simulink library "Counters_Lib"  (R2023a)
settings: Solver=ode45  StartTime=0.0  StopTime=10.0  RelTol=1e-3  EnableMultiTasking=on
libraries: simulink_extras x18, Miscellaneous x1
settings Model: Creator=Jozko Mrkvicka  LastModifiedBy=Jozko Mrkvicka
settings SolverCC: AlgebraicLoopSolver=TrustRegion
settings DataIOCC: LimitDataPoints=on  ReturnWorkspaceOutputs=off
settings OptimizationCC: LifeSpan=inf
settings DebuggingCC: UnconnectedInputMsg=warning  UnconnectedOutputMsg=warning  UnconnectedLineMsg=warning  AllowSymbolicDim=off  SFUnexpectedBacktrackingDiag=warning  SFNoUnconditionalDefaultTransitionDiag=warning  ArithmeticOperatorsInVariantConditions=warning
settings ModelReferenceCC: EnableRefExpFcnMdlSchedulingChecks=on
settings SFSimCC: SimUseLocalCustomCode=off  CustomCodeUndefinedFunction=UseInterfaceOnly
settings RTWCC: RTWUseLocalCustomCode=off
settings CodeAppCC: StateflowObjectComments=on
settings GRTTargetCC: TargetLangStandard=C89/C90 (ANSI)
settings ConfigComp: CovMetricSettings=dw  CovSaveCumulativeToWorkspaceVar=on  CovSaveSingleToWorkspaceVar=on  CovExternalEMLEnable=off

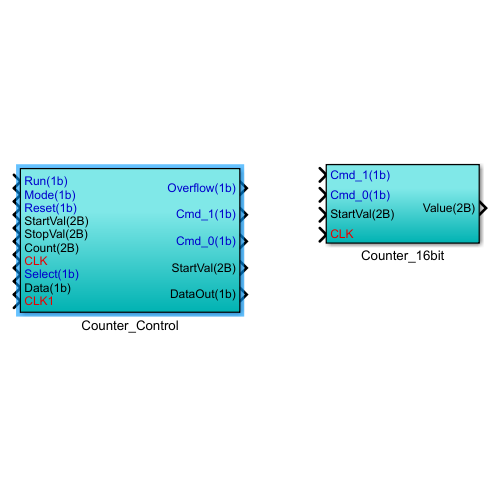
[thumbnail: Simulink's stored preview of the top-level diagram]
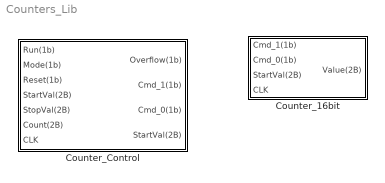
== system Counters_Lib ==
  Counter_16bit : Subsystem
  Counter_Control : Subsystem

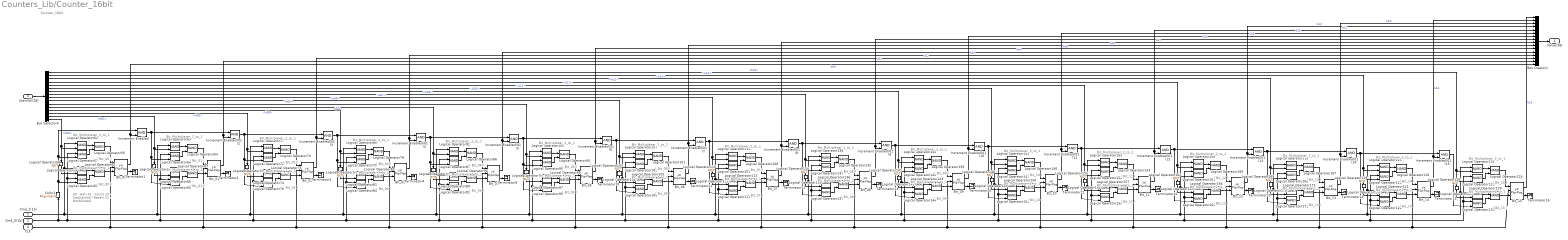
== system Counters_Lib/Counter_16bit ==
  note: Counter_16bit
  note: 00 - Halt
      | 01 - Count
      | 10 - SetStartVal (Reset)
      | 11 - NotAllowed
  note: ( Bit_00 )
  note: Bit_Multiplexer_2_to_1
  note: Bit_Multiplexer_2_to_1
  note: ( Bit_00 )
  note: ( Bit_01 )
  note: Bit_Multiplexer_2_to_1
  note: Bit_Multiplexer_2_to_1
  note: ( Bit_01 )
  note: ( Bit_02 )
  note: Bit_Multiplexer_2_to_1
  note: Bit_Multiplexer_2_to_1
  note: ( Bit_02 )
  note: ( Bit_03 )
  note: Bit_Multiplexer_2_to_1
  note: Bit_Multiplexer_2_to_1
  note: ( Bit_03 )
  note: ( Bit_04 )
  note: Bit_Multiplexer_2_to_1
  note: Bit_Multiplexer_2_to_1
  note: ( Bit_04 )
  note: ( Bit_05 )
  note: Bit_Multiplexer_2_to_1
  note: Bit_Multiplexer_2_to_1
  note: ( Bit_05 )
  note: ( Bit_06 )
  note: Bit_Multiplexer_2_to_1
  note: Bit_Multiplexer_2_to_1
  note: ( Bit_06 )
  note: ( Bit_07 )
  note: Bit_Multiplexer_2_to_1
  note: Bit_Multiplexer_2_to_1
  note: ( Bit_07 )
  note: ( Bit_11 )
  note: Bit_Multiplexer_2_to_1
  note: ( Bit_11 )
  note: ( Bit_12 )
  note: Bit_Multiplexer_2_to_1
  note: ( Bit_15 )
  note: Bit_Multiplexer_2_to_1
  note: Bit_Multiplexer_2_to_1
  note: Bit_Multiplexer_2_to_1
  note: ( Bit_14 )
  note: Bit_Multiplexer_2_to_1
  note: ( Bit_13 )
  note: ( Bit_15 )
  note: ( Bit_13 )
  note: Bit_Multiplexer_2_to_1
  note: ( Bit_14 )
  note: Bit_Multiplexer_2_to_1
  note: Bit_Multiplexer_2_to_1
  note: ( Bit_10 )
  note: ( Bit_10 )
  note: Bit_Multiplexer_2_to_1
  note: Bit_Multiplexer_2_to_1
  note: Bit_Multiplexer_2_to_1
  note: ( Bit_08 )
  note: Bit_Multiplexer_2_to_1
  note: Bit_Multiplexer_2_to_1
  note: Bit_Multiplexer_2_to_1
  note: Bit_Multiplexer_2_to_1
  note: ( Bit_08 )
  note: ( Bit_09 )
  note: ( Bit_12 )
  note: ( Bit_09 )
  Cmd_1(1b) : Inport
  Cmd_0(1b) : Inport  Port=2
  StartVal(2B) : Inport  Port=3
  CLK : Inport  Port=4
  Bit_00 : simulink_extras/Flip Flops/J-K Flip-Flop  initial_condition=0
  Bit_01 : simulink_extras/Flip Flops/J-K Flip-Flop  initial_condition=0
  Bit_02 : simulink_extras/Flip Flops/J-K Flip-Flop  initial_condition=0
  Bit_03 : simulink_extras/Flip Flops/J-K Flip-Flop  initial_condition=0
  Bit_04 : simulink_extras/Flip Flops/J-K Flip-Flop  initial_condition=0
  Bit_05 : simulink_extras/Flip Flops/J-K Flip-Flop  initial_condition=0
  Bit_06 : simulink_extras/Flip Flops/J-K Flip-Flop  initial_condition=0
  Bit_07 : simulink_extras/Flip Flops/J-K Flip-Flop  initial_condition=0
  Bit_08 : simulink_extras/Flip Flops/J-K Flip-Flop  initial_condition=0
  Bit_09 : simulink_extras/Flip Flops/J-K Flip-Flop  initial_condition=0
  Bit_{10..15} (6 alike) : simulink_extras/Flip Flops/J-K Flip-Flop  initial_condition=0
  Bus Creator1 : BusCreator  Inputs=16
  Bus Selector4 : BusSelector  OutputSignals=b15,b14,b13,b12,b11,b10,b09,b08,b07,b06,b05,b04,b03,b02,b01,b00
  Color1 : Miscellaneous/Alignment  SystemSampleTime=-1  VariantActivationTime=update diagram  Latency=0  AutoFrameSizeCalculation=off
  Increment Enabled : Logic  IconShape=distinctive  AllPortsSameDT=off  OutDataTypeStr=boolean
  Increment Enabled(01){2..15} (14 alike) : Logic  IconShape=distinctive  AllPortsSameDT=off  OutDataTypeStr=boolean
  Logical Operator{57,59,61..62,64,66,68..69,72,74,76..77,79,81,84..85,87,89,91..92,95,97,99..100,102,104,106..107,109,111,113..115,118,120,122..123,125,127,130..131,133,135,137..138,140,142,144..145,147,149,151..152,154,156,158..159,161,163,165..166,168,170,172} (64 alike) : Logic  Operator=NAND  IconShape=distinctive  AllPortsSameDT=off  OutDataTypeStr=boolean
  Logical Operator{56,60,63,67,70,75,78,83,86,90,94,98,101,105,108,112,116,121,124,129,132,136,139,143,146,150,153,157,160,164,167,171} (32 alike) : Logic  Operator=NAND  IconShape=distinctive  OutDataTypeStr=boolean
  Logical Operator{58,65,73,80,88,96,103,110,119,126,134,141,148,155,162,169} (16 alike) : Logic  Operator=NOT  IconShape=distinctive  AllPortsSameDT=off  OutDataTypeStr=boolean
  Terminator{1..4,9..16,20..23} (16 alike) : Terminator
  Value(2B) : Outport
  wires:
  Bus Selector4/16 -> Logical Operator62/2, Logical Operator58/1  "<b00>"
  CLK/1 -> Bit_00/2, Bit_01/2, Bit_02/2, Bit_03/2, Bit_04/2, Bit_05/2, Bit_06/2, Bit_07/2, Bit_08/2, Bit_09/2, Bit_10/2, Bit_11/2, Bit_12/2, Bit_13/2, Bit_15/2, Bit_14/2
  Color1/1 -> Increment Enabled/1, Logical Operator57/2, Logical Operator61/2
  Bit_00/2 -> Terminator1/1
  Cmd_1(1b)/1 -> Logical Operator59/1, Logical Operator62/1, Logical Operator66/1, Logical Operator69/1, Logical Operator74/1, Logical Operator77/1, Logical Operator81/1, Logical Operator85/1, Logical Operator89/1, Logical Operator92/1, Logical Operator97/1, Logical Operator100/1, Logical Operator104/1, Logical Operator107/1, Logical Operator111/1, Logical Operator114/1, Logical Operator135/1, Logical Operator138/1, Logical Operator142/1, Logical Operator145/1, Logical Operator149/1, Logical Operator152/1, Logical Operator156/1, Logical Operator159/1, Logical Operator163/1, Logical Operator166/1, Logical Operator170/1, Logical Operator115/1, Logical Operator120/1, Logical Operator123/1, Logical Operator127/1, Logical Operator131/1
  Logical Operator58/1 -> Logical Operator59/2
  Logical Operator57/1 -> Logical Operator56/2
  Logical Operator62/1 -> Logical Operator56/1
  Logical Operator56/1 -> Bit_00/1
  Logical Operator61/1 -> Logical Operator60/2
  Logical Operator59/1 -> Logical Operator60/1
  Logical Operator60/1 -> Bit_00/3
  Bus Selector4/15 -> Logical Operator69/2, Logical Operator65/1  "<b01>"
  Increment Enabled/1 -> Increment Enabled(01)2/1, Logical Operator64/2, Logical Operator68/2
  Bit_01/2 -> Terminator2/1
  Logical Operator65/1 -> Logical Operator66/2
  Logical Operator64/1 -> Logical Operator63/2
  Logical Operator69/1 -> Logical Operator63/1
  Logical Operator63/1 -> Bit_01/1
  Logical Operator68/1 -> Logical Operator67/2
  Logical Operator66/1 -> Logical Operator67/1
  Logical Operator67/1 -> Bit_01/3
  Bus Selector4/14 -> Logical Operator77/2, Logical Operator73/1  "<b02>"
  Increment Enabled(01)2/1 -> Increment Enabled(01)3/1, Logical Operator72/2, Logical Operator76/2
  Bit_02/2 -> Terminator3/1
  Logical Operator73/1 -> Logical Operator74/2
  Logical Operator72/1 -> Logical Operator70/2
  Logical Operator77/1 -> Logical Operator70/1
  Logical Operator70/1 -> Bit_02/1
  Logical Operator76/1 -> Logical Operator75/2
  Logical Operator74/1 -> Logical Operator75/1
  Logical Operator75/1 -> Bit_02/3
  Bus Selector4/13 -> Logical Operator85/2, Logical Operator80/1  "<b03>"
  Increment Enabled(01)3/1 -> Increment Enabled(01)4/1, Logical Operator79/2, Logical Operator84/2
  Bit_03/2 -> Terminator4/1
  Logical Operator80/1 -> Logical Operator81/2
  Logical Operator79/1 -> Logical Operator78/2
  Logical Operator85/1 -> Logical Operator78/1
  Logical Operator78/1 -> Bit_03/1
  Logical Operator84/1 -> Logical Operator83/2
  Logical Operator81/1 -> Logical Operator83/1
  Logical Operator83/1 -> Bit_03/3
  Bus Selector4/12 -> Logical Operator92/2, Logical Operator88/1  "<b04>"
  Increment Enabled(01)4/1 -> Increment Enabled(01)5/1, Logical Operator87/2, Logical Operator91/2
  Bit_04/2 -> Terminator9/1
  Logical Operator88/1 -> Logical Operator89/2
  Logical Operator87/1 -> Logical Operator86/2
  Logical Operator92/1 -> Logical Operator86/1
  Logical Operator86/1 -> Bit_04/1
  Logical Operator91/1 -> Logical Operator90/2
  Logical Operator89/1 -> Logical Operator90/1
  Logical Operator90/1 -> Bit_04/3
  Bus Selector4/11 -> Logical Operator100/2, Logical Operator96/1  "<b05>"
  Increment Enabled(01)5/1 -> Increment Enabled(01)6/1, Logical Operator95/2, Logical Operator99/2
  Bit_05/2 -> Terminator10/1
  Logical Operator96/1 -> Logical Operator97/2
  Logical Operator95/1 -> Logical Operator94/2
  Logical Operator100/1 -> Logical Operator94/1
  Logical Operator94/1 -> Bit_05/1
  Logical Operator99/1 -> Logical Operator98/2
  Logical Operator97/1 -> Logical Operator98/1
  Logical Operator98/1 -> Bit_05/3
  Bus Selector4/10 -> Logical Operator107/2, Logical Operator103/1  "<b06>"
  Increment Enabled(01)6/1 -> Increment Enabled(01)7/1, Logical Operator102/2, Logical Operator106/2
  Bit_06/2 -> Terminator11/1
  Logical Operator103/1 -> Logical Operator104/2
  Logical Operator102/1 -> Logical Operator101/2
  Logical Operator107/1 -> Logical Operator101/1
  Logical Operator101/1 -> Bit_06/1
  Logical Operator106/1 -> Logical Operator105/2
  Logical Operator104/1 -> Logical Operator105/1
  Logical Operator105/1 -> Bit_06/3
  Bus Selector4/9 -> Logical Operator114/2, Logical Operator110/1  "<b07>"
  Increment Enabled(01)7/1 -> Increment Enabled(01)8/1, Logical Operator109/2, Logical Operator113/2
  Bit_07/2 -> Terminator12/1
  Logical Operator110/1 -> Logical Operator111/2
  Logical Operator109/1 -> Logical Operator108/2
  Logical Operator114/1 -> Logical Operator108/1
  Logical Operator108/1 -> Bit_07/1
  Logical Operator113/1 -> Logical Operator112/2
  Logical Operator111/1 -> Logical Operator112/1
  Logical Operator112/1 -> Bit_07/3
  Logical Operator157/1 -> Bit_11/3
  Logical Operator156/1 -> Logical Operator157/1
  Logical Operator153/1 -> Bit_11/1
  Logical Operator155/1 -> Logical Operator156/2
  Logical Operator165/1 -> Logical Operator164/2
  Logical Operator160/1 -> Bit_12/1
  Logical Operator164/1 -> Bit_12/3
  Logical Operator163/1 -> Logical Operator164/1
  Logical Operator166/1 -> Logical Operator160/1
  Bit_12/2 -> Terminator23/1
  Bus Selector4/4 -> Logical Operator166/2, Logical Operator162/1  "<b12>"
  Increment Enabled(01)12/1 -> Increment Enabled(01)13/1, Logical Operator161/2, Logical Operator165/2
  Increment Enabled(01)13/1 -> Increment Enabled(01)14/1, Logical Operator168/2, Logical Operator172/2
  Logical Operator125/1 -> Logical Operator124/2
  Logical Operator124/1 -> Bit_15/1
  Logical Operator129/1 -> Bit_15/3
  Logical Operator127/1 -> Logical Operator129/1
  Logical Operator130/1 -> Logical Operator129/2
  Logical Operator116/1 -> Bit_14/1
  Logical Operator122/1 -> Logical Operator121/2
  Logical Operator121/1 -> Bit_14/3
  Logical Operator120/1 -> Logical Operator121/1
  Logical Operator118/1 -> Logical Operator116/2
  Logical Operator119/1 -> Logical Operator120/2
  Bit_14/2 -> Terminator15/1
  Logical Operator131/1 -> Logical Operator124/1
  Increment Enabled(01)14/1 -> Increment Enabled(01)15/1, Logical Operator118/2, Logical Operator122/2
  Cmd_0(1b)/1 -> Color1/1, Logical Operator61/1, Logical Operator57/1, Logical Operator68/1, Logical Operator64/1, Logical Operator130/1, Logical Operator125/1, Logical Operator122/1, Logical Operator118/1, Logical Operator172/1, Logical Operator168/1, Logical Operator165/1, Logical Operator161/1, Logical Operator158/1, Logical Operator154/1, Logical Operator151/1, Logical Operator147/1, Logical Operator144/1, Logical Operator140/1, Logical Operator137/1, Logical Operator133/1, Logical Operator113/1, Logical Operator109/1, Logical Operator106/1, Logical Operator102/1, Logical Operator99/1, Logical Operator95/1, Logical Operator91/1, Logical Operator87/1, Logical Operator84/1, Logical Operator79/1, Logical Operator76/1, Logical Operator72/1
  Logical Operator126/1 -> Logical Operator127/2
  Bus Selector4/2 -> Logical Operator123/2, Logical Operator119/1  "<b14>"
  Logical Operator123/1 -> Logical Operator116/1
  Increment Enabled(01)10/1 -> Increment Enabled(01)11/1, Logical Operator147/2, Logical Operator151/2
  Logical Operator170/1 -> Logical Operator171/1
  Logical Operator167/1 -> Bit_13/1
  Logical Operator169/1 -> Logical Operator170/2
  Bit_13/2 -> Terminator14/1
  Bus Selector4/5 -> Logical Operator159/2, Logical Operator155/1  "<b11>"
  Logical Operator172/1 -> Logical Operator171/2
  Logical Operator168/1 -> Logical Operator167/2
  Logical Operator162/1 -> Logical Operator163/2
  Increment Enabled(01)11/1 -> Increment Enabled(01)12/1, Logical Operator154/2, Logical Operator158/2
  Logical Operator150/1 -> Bit_10/3
  Logical Operator152/1 -> Logical Operator146/1
  Logical Operator148/1 -> Logical Operator149/2
  Logical Operator146/1 -> Bit_10/1
  Logical Operator147/1 -> Logical Operator146/2
  Logical Operator151/1 -> Logical Operator150/2
  Logical Operator149/1 -> Logical Operator150/1
  Logical Operator158/1 -> Logical Operator157/2
  Bit_10/2 -> Terminator21/1
  Logical Operator115/1 -> Logical Operator167/1
  Logical Operator135/1 -> Logical Operator136/1
  Increment Enabled(01)9/1 -> Increment Enabled(01)10/1, Logical Operator140/2, Logical Operator144/2
  Logical Operator159/1 -> Logical Operator153/1
  Logical Operator133/1 -> Logical Operator132/2
  Logical Operator132/1 -> Bit_08/1
  Logical Operator171/1 -> Bit_13/3
  Logical Operator154/1 -> Logical Operator153/2
  Increment Enabled(01)15/1 -> Logical Operator125/2, Logical Operator130/2
  Bit_08/2 -> Terminator13/1
  Increment Enabled(01)8/1 -> Increment Enabled(01)9/1, Logical Operator133/2, Logical Operator137/2
  Logical Operator134/1 -> Logical Operator135/2
  Logical Operator138/1 -> Logical Operator132/1
  Bus Selector4/8 -> Logical Operator138/2, Logical Operator134/1  "<b08>"
  Logical Operator161/1 -> Logical Operator160/2
  Logical Operator136/1 -> Bit_08/3
  Logical Operator145/1 -> Logical Operator139/1
  Logical Operator141/1 -> Logical Operator142/2
  Bus Selector4/3 -> Logical Operator115/2, Logical Operator169/1  "<b13>"
  Bit_09/2 -> Terminator20/1
  Bit_11/2 -> Terminator22/1
  Logical Operator137/1 -> Logical Operator136/2
  Bit_15/2 -> Terminator16/1
  Logical Operator140/1 -> Logical Operator139/2
  Bus Selector4/7 -> Logical Operator145/2, Logical Operator141/1  "<b09>"
  Bus Selector4/1 -> Logical Operator131/2, Logical Operator126/1  "<b15>"
  Bus Selector4/6 -> Logical Operator152/2, Logical Operator148/1  "<b10>"
  Logical Operator139/1 -> Bit_09/1
  Logical Operator143/1 -> Bit_09/3
  Logical Operator142/1 -> Logical Operator143/1
  Logical Operator144/1 -> Logical Operator143/2
  StartVal(2B)/1 -> Bus Selector4/1
  Bit_12/1 -> Bus Creator1/4, Increment Enabled(01)13/2  "b12"
  Bit_10/1 -> Bus Creator1/6, Increment Enabled(01)11/2  "b10"
  Bit_08/1 -> Bus Creator1/8, Increment Enabled(01)9/2  "b08"
  Bit_11/1 -> Bus Creator1/5, Increment Enabled(01)12/2  "b11"
  Bit_09/1 -> Bus Creator1/7, Increment Enabled(01)10/2  "b09"
  Bit_03/1 -> Bus Creator1/13, Increment Enabled(01)4/2  "b03"
  Bit_01/1 -> Bus Creator1/15, Increment Enabled(01)2/2  "b01"
  Bit_00/1 -> Bus Creator1/16, Increment Enabled/2  "b00"
  Bit_06/1 -> Bus Creator1/10, Increment Enabled(01)7/2  "b06"
  Bit_04/1 -> Bus Creator1/12, Increment Enabled(01)5/2  "b04"
  Bit_07/1 -> Bus Creator1/9, Increment Enabled(01)8/2  "b07"
  Bit_02/1 -> Bus Creator1/14, Increment Enabled(01)3/2  "b02"
  Bit_05/1 -> Bus Creator1/11, Increment Enabled(01)6/2  "b05"
  Bit_15/1 -> Bus Creator1/1  "b15"
  Bit_14/1 -> Bus Creator1/2, Increment Enabled(01)15/2  "b14"
  Bit_13/1 -> Bus Creator1/3, Increment Enabled(01)14/2  "b13"
  Bus Creator1/1 -> Value(2B)/1

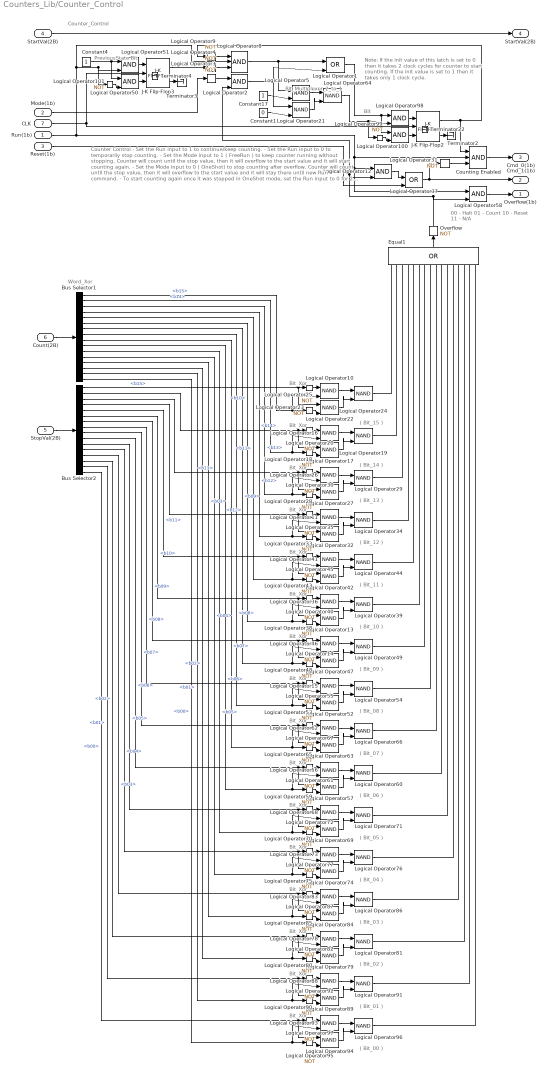
== system Counters_Lib/Counter_Control ==
  note: Counter_Control
  note: Note:
      | If the init value of this latch is set to 0 then it takes 2 clock cycles for counter to start counting.
      | If the init value is set to 1 then it takes only 1 clock cycle.
  note: 00 - Halt
      | 01 - Count
      | 10 - Reset
      | 11 - N/A
  note: Bit_Multiplexer_2_to_1
  note: Bit_Xor
  note: ( Bit_12 )
  note: Bit_Xor
  note: Bit_Xor
  note: ( Bit_01 )
  note: ( Bit_13 )
  note: ( Bit_14 )
  note: ( Bit_11 )
  note: ( Bit_00 )
  note: ( Bit_08 )
  note: ( Bit_10 )
  note: Bit_Xor
  note: Bit_Xor
  note: ( Bit_09 )
  note: Word_Xor
  note: Bit_Xor
  note: Bit_Xor
  note: Bit_Xor
  note: Bit_Xor
  note: ( Bit_03 )
  note: Bit_Xor
  note: ( Bit_15 )
  note: ( Bit_04 )
  note: Bit_Xor
  note: ( Bit_02 )
  note: Bit_Xor
  note: ( Bit_06 )
  note: Bit_Xor
  note: ( Bit_07 )
  note: ( Bit_05 )
  note: Bit_Xor
  note: Bit_Xor
  note: Bit_Xor
  note: Counter Control
      |
      | - Set the Run input to 1 to continue/keep counting.
      | - Set the Run input to 0 to temporarily stop counting.
      |
      | - Set the Mode input to 1 ( FreeRun ) to keep counter running without stopping. Counter will count until the stop value, then it will overflow to the start value and it will start counting again.
      |
      | - Set the Mode input to 0 ( OneShot) to stop counting after overflow. Counter will count until the stop value, then it will overflow to the start value and it will stay there until new Run command.
      |
      | - To start counting again once it was stopped in OneShot mode, set the Run input to 0 for 2 clock cycles and then set it back to 1 .
      |
      | - Set the Reset input to 1 :
      | - to configure new start value,
      | - to reset counter to its preconfigured start value.
  note: Bit
  note: PreviousState Bit
  Run(1b) : Inport
  Mode(1b) : Inport  Port=2
  Reset(1b) : Inport  Port=3
  StartVal(2B) : Inport  Port=4
  StopVal(2B) : Inport  Port=5
  Count(2B) : Inport  Port=6
  CLK : Inport  Port=7
  Bus Selector1 : BusSelector  OutputSignals=b15,b14,b13,b12,b11,b10,b09,b08,b07,b06,b05,b04,b03,b02,b01,b00
  Bus Selector2 : BusSelector  OutputSignals=b15,b14,b13,b12,b11,b10,b09,b08,b07,b06,b05,b04,b03,b02,b01,b00
  Constant1 : Constant  Value=0  OutDataTypeStr=boolean
  Constant17 : Constant  OutDataTypeStr=boolean
  Constant4 : Constant  OutDataTypeStr=boolean
  Counting Enabled : Logic  Inputs=3  IconShape=distinctive  AllPortsSameDT=off  OutDataTypeStr=boolean
  Equal1 : Logic  Operator=OR  Inputs=16  IconShape=distinctive  AllPortsSameDT=off  OutDataTypeStr=boolean
  J-K Flip-Flop2 : simulink_extras/Flip Flops/J-K Flip-Flop  initial_condition=0
  J-K Flip-Flop3 : simulink_extras/Flip Flops/J-K Flip-Flop  initial_condition=0
  Logical Operator1 : Logic  Operator=OR  IconShape=distinctive  AllPortsSameDT=off  OutDataTypeStr=boolean
  Logical Operator{5,10..11,13,15..17,19,21..22,24,26..27,29,32,34,36,39,41..42,44,46..47,49,52,54,56..57,60,62..63,66,68..69,71,73..74,76,78..79,81,83..84,86,88..89,91,93..94,96} (50 alike) : Logic  Operator=NAND  IconShape=distinctive  AllPortsSameDT=off  OutDataTypeStr=boolean
  Logical Operator{2,12,50..51,58,98,100} (7 alike) : Logic  IconShape=distinctive  AllPortsSameDT=off  OutDataTypeStr=boolean
  Logical Operator{14,18,20,23,25,28,30,33,35,38,40,43,45,48,53,55,59,61,65,67,70,72,75,77,80,82,85,87,90,92,95,97,99,101} (34 alike) : Logic  Operator=NOT  IconShape=distinctive  AllPortsSameDT=off  OutDataTypeStr=boolean
  Logical Operator{3..4,9,31} (4 alike) : Logic  Operator=NOT  Inputs=4  IconShape=distinctive  AllPortsSameDT=off  OutDataTypeStr=boolean
  Logical Operator37 : Logic  Operator=OR  IconShape=distinctive  AllPortsSameDT=off  OutDataTypeStr=boolean
  Logical Operator64 : Logic  Operator=NAND  IconShape=distinctive  OutDataTypeStr=boolean
  Logical Operator8 : Logic  Inputs=3  IconShape=distinctive  AllPortsSameDT=off  OutDataTypeStr=boolean
  Overflow : Logic  Operator=NOT  IconShape=distinctive  AllPortsSameDT=off  OutDataTypeStr=boolean
  Terminator{2..4,22} (4 alike) : Terminator
  Overflow(1b) : Outport
  Cmd_1(1b) : Outport  Port=2
  Cmd_0(1b) : Outport  Port=3
  " StartVal(2B)" : Outport  Port=4
  wires:
  Logical Operator31/1 -> Counting Enabled/3
  Constant1/1 -> Logical Operator21/2
  Mode(1b)/1 -> Logical Operator3/1
  Logical Operator37/1 -> Logical Operator31/1, Cmd_1(1b)/1
  Logical Operator4/1 -> Logical Operator8/3
  Overflow/1 -> Logical Operator58/2, Logical Operator12/2, Logical Operator2/2
  Logical Operator3/1 -> Logical Operator2/1
  Constant17/1 -> Logical Operator5/2
  Logical Operator8/1 -> Logical Operator1/1, Logical Operator5/1
  Logical Operator9/1 -> Logical Operator8/1
  Logical Operator2/1 -> Logical Operator21/1, Logical Operator1/2
  Logical Operator12/1 -> Logical Operator37/1
  J-K Flip-Flop2/1 -> Logical Operator9/1, Counting Enabled/1
  Counting Enabled/1 -> Cmd_0(1b)/1
  Reset(1b)/1 -> Logical Operator37/2
  Equal1/1 -> Overflow/1
  StartVal(2B)/1 -> " StartVal(2B)"/1
  Logical Operator21/1 -> Logical Operator64/2
  Logical Operator5/1 -> Logical Operator64/1
  Logical Operator24/1 -> Equal1/1
  Logical Operator85/1 -> Logical Operator84/2
  Logical Operator57/1 -> Logical Operator60/2
  Bus Selector2/15 -> Logical Operator92/1, Logical Operator89/1  "<b01>"
  Logical Operator28/1 -> Logical Operator27/2
  Logical Operator63/1 -> Logical Operator66/2
  Logical Operator97/1 -> Logical Operator93/1
  Logical Operator73/1 -> Logical Operator76/1
  Bus Selector2/12 -> Logical Operator77/1, Logical Operator74/1  "<b04>"
  Logical Operator61/1 -> Logical Operator56/1
  Bus Selector1/10 -> Logical Operator56/2, Logical Operator59/1  "<b06>"
  Bus Selector2/1 -> Logical Operator25/1, Logical Operator22/1  "<b15>"
  Logical Operator84/1 -> Logical Operator86/2
  Logical Operator41/1 -> Logical Operator44/1
  Logical Operator96/1 -> Equal1/16
  Logical Operator53/1 -> Logical Operator52/2
  Logical Operator79/1 -> Logical Operator81/2
  Logical Operator95/1 -> Logical Operator94/2
  Logical Operator80/1 -> Logical Operator79/2
  Logical Operator91/1 -> Equal1/15
  Logical Operator76/1 -> Equal1/12
  Logical Operator90/1 -> Logical Operator89/2
  Logical Operator78/1 -> Logical Operator81/1
  Logical Operator92/1 -> Logical Operator88/1
  Bus Selector1/13 -> Logical Operator83/2, Logical Operator85/1  "<b03>"
  Bus Selector1/15 -> Logical Operator88/2, Logical Operator90/1  "<b01>"
  Logical Operator88/1 -> Logical Operator91/1
  Bus Selector2/13 -> Logical Operator87/1, Logical Operator84/1  "<b03>"
  Logical Operator43/1 -> Logical Operator42/2
  Logical Operator87/1 -> Logical Operator83/1
  Logical Operator32/1 -> Logical Operator34/2
  Logical Operator46/1 -> Logical Operator49/1
  Logical Operator48/1 -> Logical Operator47/2
  Bus Selector1/6 -> Logical Operator36/2, Logical Operator38/1  "<b10>"
  Logical Operator94/1 -> Logical Operator96/2
  Logical Operator39/1 -> Equal1/6
  Bus Selector1/8 -> Logical Operator15/2, Logical Operator53/1  "<b08>"
  Logical Operator44/1 -> Equal1/5
  Logical Operator55/1 -> Logical Operator15/1
  Logical Operator42/1 -> Logical Operator44/2
  Logical Operator14/1 -> Logical Operator46/1
  Logical Operator40/1 -> Logical Operator36/1
  Logical Operator54/1 -> Equal1/8
  Logical Operator52/1 -> Logical Operator54/2
  Logical Operator45/1 -> Logical Operator41/1
  Logical Operator11/1 -> Logical Operator34/1
  Logical Operator33/1 -> Logical Operator32/2
  Logical Operator10/1 -> Logical Operator24/1
  Logical Operator15/1 -> Logical Operator54/1
  Bus Selector2/4 -> Logical Operator35/1, Logical Operator32/1  "<b12>"
  Bus Selector2/2 -> Logical Operator20/1, Logical Operator17/1  "<b14>"
  Logical Operator26/1 -> Logical Operator29/1
  Bus Selector2/7 -> Logical Operator14/1, Logical Operator47/1  "<b09>"
  Logical Operator18/1 -> Logical Operator17/2
  Logical Operator20/1 -> Logical Operator16/1
  Logical Operator19/1 -> Equal1/2
  Logical Operator22/1 -> Logical Operator24/2
  Logical Operator17/1 -> Logical Operator19/2
  Logical Operator25/1 -> Logical Operator10/1
  Logical Operator16/1 -> Logical Operator19/1
  Logical Operator67/1 -> Logical Operator62/1
  Bus Selector1/16 -> Logical Operator93/2, Logical Operator95/1  "<b00>"
  StopVal(2B)/1 -> Bus Selector2/1
  Count(2B)/1 -> Bus Selector1/1
  Logical Operator75/1 -> Logical Operator74/2
  Logical Operator70/1 -> Logical Operator69/2
  Bus Selector1/4 -> Logical Operator11/2, Logical Operator33/1  "<b12>"
  Bus Selector1/3 -> Logical Operator26/2, Logical Operator28/1  "<b13>"
  Bus Selector1/7 -> Logical Operator46/2, Logical Operator48/1  "<b09>"
  Bus Selector2/14 -> Logical Operator82/1, Logical Operator79/1  "<b02>"
  Logical Operator29/1 -> Equal1/3
  Logical Operator38/1 -> Logical Operator13/2
  Bus Selector2/11 -> Logical Operator72/1, Logical Operator69/1  "<b05>"
  Bus Selector1/1 -> Logical Operator10/2, Logical Operator23/1  "<b15>"
  Logical Operator69/1 -> Logical Operator71/2
  Logical Operator47/1 -> Logical Operator49/2
  Logical Operator86/1 -> Equal1/13
  Bus Selector2/8 -> Logical Operator55/1, Logical Operator52/1  "<b08>"
  Bus Selector1/2 -> Logical Operator16/2, Logical Operator18/1  "<b14>"
  Logical Operator83/1 -> Logical Operator86/1
  Logical Operator59/1 -> Logical Operator57/2
  Bus Selector1/11 -> Logical Operator68/2, Logical Operator70/1  "<b05>"
  Bus Selector2/3 -> Logical Operator30/1, Logical Operator27/1  "<b13>"
  Bus Selector2/10 -> Logical Operator61/1, Logical Operator57/1  "<b06>"
  Logical Operator34/1 -> Equal1/4
  Logical Operator30/1 -> Logical Operator26/1
  Logical Operator60/1 -> Equal1/10
  Bus Selector1/12 -> Logical Operator73/2, Logical Operator75/1  "<b04>"
  Logical Operator71/1 -> Equal1/11
  Logical Operator23/1 -> Logical Operator22/2
  Logical Operator36/1 -> Logical Operator39/1
  Logical Operator68/1 -> Logical Operator71/1
  Logical Operator77/1 -> Logical Operator73/1
  Logical Operator81/1 -> Equal1/14
  Logical Operator62/1 -> Logical Operator66/1
  Logical Operator35/1 -> Logical Operator11/1
  Logical Operator82/1 -> Logical Operator78/1
  Bus Selector1/9 -> Logical Operator62/2, Logical Operator65/1  "<b07>"
  Bus Selector2/6 -> Logical Operator40/1, Logical Operator13/1  "<b10>"
  Logical Operator65/1 -> Logical Operator63/2
  Logical Operator74/1 -> Logical Operator76/2
  Logical Operator49/1 -> Equal1/7
  Logical Operator66/1 -> Equal1/9
  Bus Selector2/9 -> Logical Operator67/1, Logical Operator63/1  "<b07>"
  Logical Operator93/1 -> Logical Operator96/1
  Bus Selector2/16 -> Logical Operator97/1, Logical Operator94/1  "<b00>"
  Logical Operator56/1 -> Logical Operator60/1
  Bus Selector1/14 -> Logical Operator78/2, Logical Operator80/1  "<b02>"
  Bus Selector1/5 -> Logical Operator41/2, Logical Operator43/1  "<b11>"
  Logical Operator27/1 -> Logical Operator29/2
  Logical Operator89/1 -> Logical Operator91/2
  Bus Selector2/5 -> Logical Operator45/1, Logical Operator42/1  "<b11>"
  Logical Operator72/1 -> Logical Operator68/1
  Logical Operator13/1 -> Logical Operator39/2
  Logical Operator58/1 -> Overflow(1b)/1
  Logical Operator98/1 -> J-K Flip-Flop2/1
  Logical Operator100/1 -> J-K Flip-Flop2/3
  Logical Operator64/1 -> Logical Operator99/1, Logical Operator98/2
  J-K Flip-Flop2/2 -> Terminator2/1
  CLK/1 -> J-K Flip-Flop2/2, J-K Flip-Flop3/2
  Logical Operator1/1 -> Logical Operator100/1, Logical Operator98/1
  Logical Operator99/1 -> Logical Operator100/2
  Logical Operator101/1 -> Logical Operator50/2
  Constant4/1 -> Logical Operator51/1, Logical Operator50/1
  Run(1b)/1 -> Counting Enabled/2, Logical Operator12/1, Logical Operator58/1, Logical Operator8/2, Logical Operator101/1, Logical Operator51/2
  Logical Operator51/1 -> J-K Flip-Flop3/1
  Logical Operator50/1 -> J-K Flip-Flop3/3
  J-K Flip-Flop3/2 -> Terminator3/1
  J-K Flip-Flop3/1 -> Logical Operator4/1
